simulink library "LopesDevelopmentLibrary"  (R2015b)
settings: Solver=ode45  StartTime=0.0  StopTime=10.0  RelTol=1e-3
values from neighbouring files (symbols this model uses):
  d2r = @(d) d*(pi/180)    [LopesDevelopmentLibrary_LoadParameters.m]
  ts = LopesParams.ts    [LopesDevelopmentLibrary_LoadParameters.m]
undefined symbols (not defined in the file or in its folder): anyParameterChanged, DiscIntNeverNeededParam, gcbh, LHF, LKF, LopesParams, macaddr, mxpcnetworkconfig, mxpcrtudprx, mxpcrtudptx, patientParametersChanged, port, PX, PZ, RHF, RKF, SelectorLOPESInSize, StrideTime_s, Time
undefined symbols (not defined in the file): LopesParamsSendDataArrayLen
libraries: LopesDevelopmentLibrary x288, simulink x98, dspmtrx3 x47, xpciplib x6, xpcnetworkbufferlib x5, dspsigops x4, dspstat3 x3, xpcethernetlib x2, visionstatistics x2, xpcseriallib x2, nmc x1, simulink_extras x1
(part 12 of 12)

== matlab function LopesDevelopmentLibrary/BlocksForInternalUse/GaitGenerationStartStop/OrderKeyEventsAddOne/SortAndAddKeyEvents ==
  data: kE input; kE_out output; Error output double; jointNumber input double; phase input; yy input; dydx input
function [kE_out, Error]= fcn(kE, jointNumber, phase, yy, dydx)
%#codegen
%
% This function does 5 things:
% 1. It adds the [phase; yy; dydx] to the key Events
% 2. It does keyEventPhases mod 100 (so that they're in the range [0,100)].
% 3. It checks whether the key events (after wrapping around 100) are
%    strictly increasing. If not, it generates an Exception.
%    Note that it is allowed that the key event with the lowest phase
%    is somewhere in the middle, e.g. [50, 66, 95, 101, 7, 20]' as the
%    first column is valid.
% 4. It sorts the key events such that they are strictly increasing (if
%    there are two key events at the same place, the 'first' is decreased a
%    tiny little bit (1e-10) in order to make sure they are strictly
%    increasing again. This whole step is always done, even if an exception
%    was generated.
%
% The underlying reasons:
% 1. If the key events are not in the right order, this is most probably not
%    what we want, so we should stop the whole thing.
% 2. The blocks further on in the data path require a strictly incrasing
%    key event matrix. In order to guarantee that these blocks don't crash,
%    we will make sure that they get what they want, even if the resulting
%    data would not be what we want. The exception can be used to detect
%    this situation, and at least the application does not crash.
%
% Example:
%      [  50   101   102   103 ]
%      [  66   201   202   203 ] 
%      [  95   301   302   303 ]
%  In: [ 101   401   402   403 ]
%      [   7   501   502   503 ]
%      [  20   601   602   603 ]
%  

%% Add key events
kE(mod(kE(:,1),100)==mod(phase,100),1) = kE(mod(kE(:,1),100)==mod(phase,100),1) + 1E-10;
kE2 = zeros(size(kE,1)+1,size(kE,2)); 
kE2(:,:) = [kE(kE(:,1) < phase,:);phase yy dydx;kE(kE(:,1) > phase,:)];

% Get phase data and wrap them
firstColumn = mod(kE2(:,1),100);
kE2 (:,1) = firstColumn;

% Strict increasingness can be checked by getting the diff of the phase
% data; there should be only one value <=0
nNonPositives = sum(diff([firstColumn;firstColumn(1)]) <=0);

% Exception handling
if (nNonPositives~=1),
    % Then the key events are not in correct order
    Error=jointNumber;
else
    % No error
    Error=0;
end;

while true
    % Sort them (no guarantee on identicity of two adjacent key events
    kE2 = sortrows(kE2,1);

    % Check if we have multiple key events at one spot
    firstColumn = kE2(:,1);
    d = diff(firstColumn);
    if (all(d~=0)), break; end; % Then there are no overlaps
    firstColumn(d==0) = mod(firstColumn(d==0)-1E-10,100);
    kE2(:,1) = firstColumn;
end;

kE_out = kE2;

== matlab function LopesDevelopmentLibrary/BlocksForInternalUse/GaitGenerationStartStop/AddUselessKE/AddUselessKE ==
  data: kE input; kE_out output; breaks input double
function kE_out = fcn(kE, breaks)
%#codegen
%
% This function adds several useless Ke to the keyevents
% The underlying reasons is that by doing this, KE for starting up are as
% long as KE of normal walking

% PreAllocating
kE2 = zeros(size(breaks,1)-2,3);

% Counting needed points
Npoints = size(kE2,1) - size(kE,1);

if Npoints > 0
    % Making full matrix with kE (including useless ones)
    % Useless ones are made by copying first row
    kE2(:,:) = [ones(Npoints,1)*kE(1,:);kE];
    
    % Removing 1E-10 to subsecuent points
    kE2(1:Npoints,1) = kE2(1:Npoints,1) + [Npoints:-1:1]'*-1E-10;
elseif Npoints == 0
    %In case of equal size
    kE2(:,:) = kE;
end

%% Output
kE_out = kE2;
end

== matlab function LopesDevelopmentLibrary/BlocksForInternalUse/GaitGenerationStartStop/AddUselessKEValue/AddUselessKE ==
  data: kE input; kE_out output
function kE_out = fcn(kE)
%#codegen
%
% This function adds several useless Ke to the keyevents
% The underlying reasons is that by doing this, KE for starting up are as
% long as KE of normal walking

% PreAllocating
kE2 = zeros(size(kE,1)+1,3);

% Counting needed points
Npoints = 1;

% Making full matrix with kE (including useless ones)
% Useless ones are made by copying first row
kE2(:,:) = [ones(Npoints,1)*kE(1,:);kE];

% Adding 1E-10 to subsecuent points
kE2(2:Npoints+1,1) = kE2(2:Npoints+1,1) + [1:Npoints]'*1E-10;


%% Output
kE_out = kE2;

== matlab function LopesDevelopmentLibrary/GaitGenerationExtra/VelocityHold/KeepVelo ==
  data: InputState input; SetState input; VeloIn input; LowerBound input; VeloOut output
function VeloOut = GetLowerBound(InputState,SetState,VeloIn,LowerBound)
%#codegen
% This script keeps the Velocity Constant At A Certain Level Before the
% Stopping Phase is Reached. This makes sure slowing down is always from
% the same velocity

VeloOut = 0; 

if (InputState == 3) && (SetState ~= 301 &&  SetState ~= 302 && SetState ~= 401 && SetState ~= 402)
    VeloOut(:) = LowerBound;
elseif SetState == 301 ||  SetState == 302
    VeloOut(:) = 0; 
else
    VeloOut(:) = VeloIn; 
end
end

== matlab function LopesDevelopmentLibrary/Robot control blocks/ToLopes/makeCreateSpringSpring ==
  data: normalBool input; bool output boolean; force input double
function bool  = makeBool(normalBool, force)
%#codegen

% Passes normalBool if force is -1; otherwise it forces the output
% to be equal to forceBool. In diagram:
%
% force     | normalBool || Output
% --------------------------------
%     -1    |   false    || false
%     -1    |   true     || true
%      0    |  dont'care || false
% otherwise |  dont'care || true

if force==-1
    bool = normalBool;
elseif force == 0
    bool = false;
else
    bool = true;
end;

== matlab function LopesDevelopmentLibrary/Various/RateLimiterWithReset/RateLimiterWithReset ==
  data: u input; y output; rate input; initialValue input; reset_high_active input; ts parameter; y_is_u output double
function [y,y_is_u] = RateLimiterWithReset(u, rate, initialValue, reset_high_active, ts)
%#codegen

% Note: rate should be positive!

persistent currentValue;

if isempty(currentValue)
    currentValue = initialValue;
end;

% For safety, prevent negative rate (if the rate is negative, signals grow
% out of bounds; it is better to set the rate to 0 in those cases, which
% will keep the signals fixed. Not what we want, but not dangerous either).
if rate<0,
    rate = 0;
end;

if reset_high_active,
    currentValue = initialValue;
else
    % Rate-limit
    if currentValue < u,
        currentValue = min(currentValue + rate*ts, u);
    elseif currentValue > u,
        currentValue = max(currentValue - rate*ts, u);
    %else
        % currentValue is alreay equal to u, so don't do anything
    end;
end;
y = currentValue;

if y == u,
    y_is_u = 1;
else
    y_is_u = 0;
end;

== matlab function LopesDevelopmentLibrary/StringFunctions/PadStrAsDouble/pad ==
  data: s input uint8; outArrayLen parameter; y output uint8; y_len output
function [y,y_len]= pad(s,outArrayLen)
%#codegen

% Given s, being an any-(fixed!)-length uint8-array, it outputs
% a 'string' array consisting of a default size (outArrayLen, as a
% parameter),padded with zero's
% together with a length indicating the number of 'valid' bytes in the
% string.
%
% If the string s is too long, it will use the first outputLen-1 chars (and
% add a null-char to fill the whole string up).

y = uint8(zeros(1,outArrayLen));
y_len = min(length(s), outArrayLen-1);
for i=1:y_len,
    y(i) = s(i);
end;
